simulink model "propeller"  (R2016a)
settings: Solver=VariableStepAuto  StartTime=0.0  StopTime=10.0  RelTol=1e-3
undefined symbols (not defined in the file or in its folder): magnitude
settings Model: Creator=Shahin  LastModifiedBy=Shahin

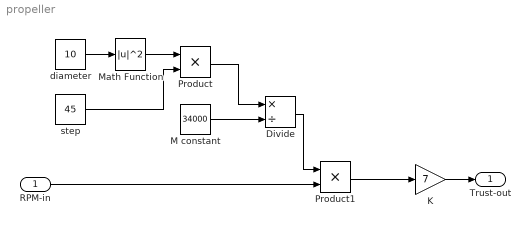
== system propeller ==
  "RPM-in " : Inport
  Divide : Product  Inputs=*/
  K : Gain  Gain=7
  M constant : Constant  Value=34000
  Math Function : Math  Operator=magnitude^2  OutputSignalType=real  SaturateOnIntegerOverflow=on
  Product : Product
  Product1 : Product
  diameter : Constant  Value=10
  step : Constant  Value=45
  Trust-out : Outport
  wires:
  diameter/1 -> Math Function/1
  step/1 -> Product/2
  Math Function/1 -> Product/1
  Product/1 -> Divide/1
  M constant/1 -> Divide/2
  Divide/1 -> Product1/1
  "RPM-in "/1 -> Product1/2
  Product1/1 -> K/1
  K/1 -> Trust-out/1
